simulink model "simLink_line"  (R2022b)
settings: Solver=FixedStepAuto  StartTime=0.0  StopTime=30  FixedStep=0.1  RelTol=1e-3
values from neighbouring files (symbols this model uses):
  length_body = pixel_body/pixel_conversion    (= 80)    [startSim.m]
  spacing = 2/pixel_conversion    (= 20)    [startSim.m]
undefined symbols (not defined in the file or in its folder): img, offset_x, offset_y, pixel, v1, v2
libraries: slpidlib x1, robotmobilelib x1
settings Model: Creator=andre  LastModifiedBy=andre

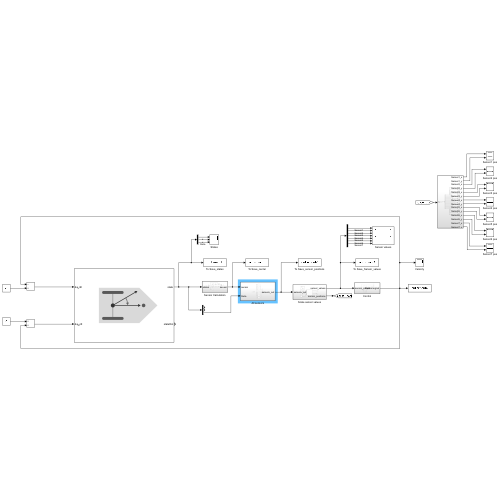
[thumbnail: Simulink's stored preview of the top-level diagram]
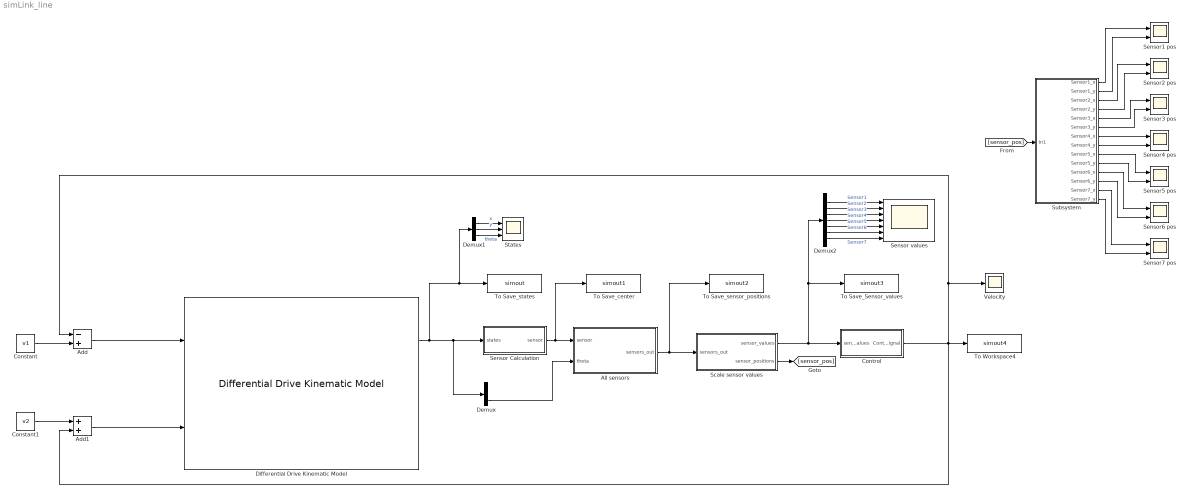
== system simLink_line ==
  Add : Sum  Inputs=-+
  Add1 : Sum
  All sensors : Subsystem
  Constant : Constant  Value=v1
  Constant1 : Constant  Value=v2
  Control : Subsystem
  Demux : Demux  Outputs=3
  Demux1 : Demux  Outputs=3
  Demux2 : Demux  Outputs=7
  Differential Drive Kinematic Model : robotmobilelib/Differential Drive Kinematic Model  VehicleInputs=Wheel Speeds  WheelRadius=0.5  WheelSpeedRange=[-inf inf]  TrackWidth=1  InitialState=initialState  SimulateUsing=Interpreted execution
  Scale sensor values : Subsystem
  Sensor Calculation : Subsystem
  Sensor values : Scope  NumInputPorts=7
  Sensor1 pos : Scope  NumInputPorts=2
  Sensor2 pos : Scope  NumInputPorts=2
  Sensor3 pos : Scope  NumInputPorts=2
  Sensor4 pos : Scope  NumInputPorts=2
  Sensor5 pos : Scope  NumInputPorts=2
  Sensor6 pos : Scope  NumInputPorts=2
  Sensor7 pos : Scope  NumInputPorts=2
  States : Scope  NumInputPorts=3
  Subsystem : Subsystem
  To Save_Sensor_values : ToWorkspace  VariableName=simout3  SaveFormat=Structure With Time  SampleTime=-1
  To Save_center : ToWorkspace  VariableName=simout1  SaveFormat=Structure With Time  SampleTime=-1
  To Save_sensor_positions : ToWorkspace  VariableName=simout2  SaveFormat=Structure With Time  SampleTime=-1
  To Save_states : ToWorkspace  VariableName=simout  SaveFormat=Structure With Time  SampleTime=-1
  To Workspace4 : ToWorkspace  VariableName=simout4  SaveFormat=Structure With Time  SampleTime=-1
  Velocity : Scope
  wires:
  Sensor Calculation/1(sensor) -> To Save_center/1, All sensors/1(sensor)
  Differential Drive Kinematic Model/1 -> Demux1/1, To Save_states/1, Demux/1, Sensor Calculation/1(states)
  All sensors/1(sensors_out) -> To Save_sensor_positions/1, Scale sensor values/1(sensors_out)
  Demux/3 -> All sensors/2(theta)
  Control/1(Control signal) -> Add1/2, To Workspace4/1, Add/1, Velocity/1
  Constant/1 -> Add/2
  Constant1/1 -> Add1/1
  Add1/1 -> Differential Drive Kinematic Model/2
  Add/1 -> Differential Drive Kinematic Model/1
  Demux1/1 -> States/1  "x"
  Demux1/2 -> States/2  "y"
  Demux1/3 -> States/3  "theta"
  Scale sensor values/1(sensor_values) -> Demux2/1, To Save_Sensor_values/1, Control/1(sensor_values)
  Demux2/1 -> Sensor values/1  "Sensor1"
  Demux2/2 -> Sensor values/2  "Sensor2"
  Demux2/3 -> Sensor values/3  "Sensor3"
  Demux2/4 -> Sensor values/4  "Sensor4"
  Demux2/5 -> Sensor values/5  "Sensor5"
  Demux2/6 -> Sensor values/6  "Sensor6"
  Demux2/7 -> Sensor values/7  "Sensor7"
  [sensor_pos] -> Subsystem/1(In1)
  Subsystem/1(Sensor1_x) -> Sensor1 pos/1
  Subsystem/2(Sensor1_y) -> Sensor1 pos/2
  Subsystem/3(Sensor2_x) -> Sensor2 pos/1
  Subsystem/4(Sensor2_y) -> Sensor2 pos/2
  Subsystem/5(Sensor3_x) -> Sensor3 pos/1
  Subsystem/6(Sensor3_y) -> Sensor3 pos/2
  Subsystem/7(Sensor4_x) -> Sensor4 pos/1
  Subsystem/8(Sensor4_y) -> Sensor4 pos/2
  Subsystem/9(Sensor5_x) -> Sensor5 pos/1
  Subsystem/10(Sensor5_y) -> Sensor5 pos/2
  Subsystem/11(Sensor6_x) -> Sensor6 pos/1
  Subsystem/12(Sensor6_y) -> Sensor6 pos/2
  Subsystem/13(Sensor7_x) -> Sensor7 pos/1
  Subsystem/14(Sensor7_y) -> Sensor7 pos/2
  Scale sensor values/2(sensor_positions) -> [sensor_pos]

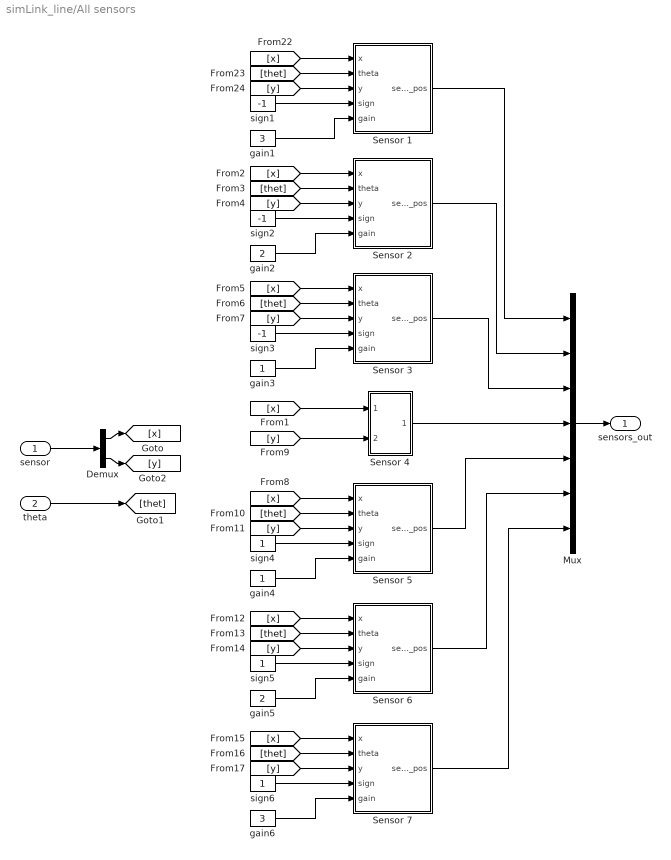
== system simLink_line/All sensors ==
  sensor : Inport
  theta : Inport  Port=2
  Demux : Demux  Outputs=2
  Mux : Mux  Inputs=7
  Sensor 1 : Subsystem
  Sensor 2 : Subsystem
  Sensor 3 : Subsystem
  Sensor 4 : Subsystem
  Sensor 5 : Subsystem
  Sensor 6 : Subsystem
  Sensor 7 : Subsystem
  gain1 : Constant  Value=3
  gain2 : Constant  Value=2
  gain3 : Constant
  gain4 : Constant
  gain5 : Constant  Value=2
  gain6 : Constant  Value=3
  sign1 : Constant  Value=-1
  sign2 : Constant  Value=-1
  sign3 : Constant  Value=-1
  sign4 : Constant
  sign5 : Constant
  sign6 : Constant
  sensors_out : Outport
  wires:
  sensor/1 -> Demux/1
  Demux/1 -> [x]
  theta/1 -> [thet]
  Demux/2 -> [y]
  Mux/1 -> sensors_out/1
  [x] -> Sensor 1/1(x)
  [thet] -> Sensor 1/2(theta)
  [y] -> Sensor 1/3(y)
  Sensor 1/1(sensor_pos) -> Mux/1
  [x] -> Sensor 4/1(In1)
  [y] -> Sensor 4/2(In2)
  Sensor 4/1(Out1) -> Mux/4
  sign1/1 -> Sensor 1/4(sign)
  gain1/1 -> Sensor 1/5(gain)
  [x] -> Sensor 2/1(x)
  [x] -> Sensor 3/1(x)
  [x] -> Sensor 5/1(x)
  [thet] -> Sensor 5/2(theta)
  [x] -> Sensor 6/1(x)
  [x] -> Sensor 7/1(x)
  Sensor 2/1(sensor_pos) -> Mux/2
  Sensor 3/1(sensor_pos) -> Mux/3
  Sensor 5/1(sensor_pos) -> Mux/5
  Sensor 6/1(sensor_pos) -> Mux/6
  Sensor 7/1(sensor_pos) -> Mux/7
  [thet] -> Sensor 2/2(theta)
  [y] -> Sensor 2/3(y)
  sign2/1 -> Sensor 2/4(sign)
  gain2/1 -> Sensor 2/5(gain)
  [thet] -> Sensor 3/2(theta)
  [y] -> Sensor 3/3(y)
  gain3/1 -> Sensor 3/5(gain)
  sign3/1 -> Sensor 3/4(sign)
  [y] -> Sensor 5/3(y)
  sign4/1 -> Sensor 5/4(sign)
  gain4/1 -> Sensor 5/5(gain)
  [thet] -> Sensor 6/2(theta)
  [y] -> Sensor 6/3(y)
  sign5/1 -> Sensor 6/4(sign)
  gain5/1 -> Sensor 6/5(gain)
  [thet] -> Sensor 7/2(theta)
  [y] -> Sensor 7/3(y)
  sign6/1 -> Sensor 7/4(sign)
  gain6/1 -> Sensor 7/5(gain)

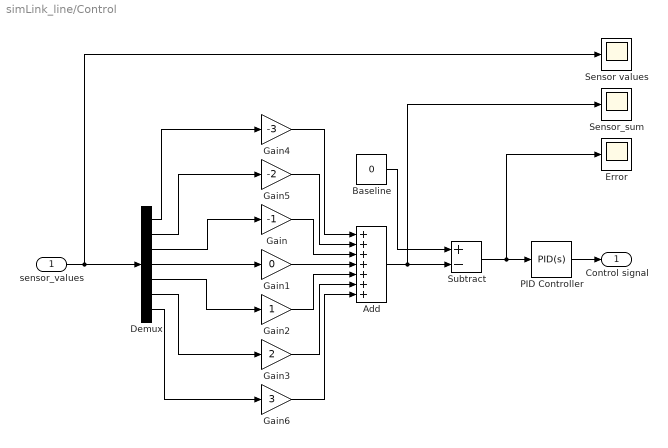
== system simLink_line/Control ==
  sensor_values : Inport
  Add : Sum  Inputs=+++++++
  Baseline : Constant  Value=0
  Demux : Demux  Outputs=7
  Error : Scope
  Gain : Gain  Gain=-1
  Gain1 : Gain  Gain=0
  Gain2 : Gain
  Gain3 : Gain  Gain=2
  Gain4 : Gain  Gain=-3
  Gain5 : Gain  Gain=-2
  Gain6 : Gain  Gain=3
  PID Controller : slpidlib/PID Controller  Controller=PID  Form=Parallel  TimeDomain=Continuous-time  UseExternalTs=off  SampleTime=-1  IntegratorMethod=Forward Euler  FilterMethod=Forward Euler  ControllerParametersSource=internal  P=0.01  I=1  UseKiTs=off  D=0  N=100  UseFilter=on  TunerSelectOption=Transfer Function Based (PID Tuner App)  InitialConditionSource=internal  InitialConditionForIntegrator=0  InitialConditionForFilter=0  DifferentiatorICPrevScaledInput=0  ExternalReset=none  TrackingMode=off  Kt=1  LimitOutput=off  SatLimitsSource=internal  UpperSaturationLimit=inf  LowerSaturationLimit=-inf  LinearizeAsGain=on  AntiWindupMode=none  Kb=1  LimitIntegrator=off  UpperIntegratorSaturationLimit=inf  LowerIntegratorSaturationLimit=-inf  POutMin=[]  POutMax=[]  IOutMin=[]  IOutMax=[]  DOutMin=[]  DOutMax=[]  NOutMin=[]  NOutMax=[]  SumOutMin=[]  SumOutMax=[]  SaturationOutMin=[]  SaturationOutMax=[]  PParamMin=[]  PParamMax=[]  IParamMin=[]  IParamMax=[]  DParamMin=[]  DParamMax=[]  NParamMin=[]  NParamMax=[]  KbParamMin=[]  KbParamMax=[]  KtParamMin=[]  KtParamMax=[]  KbOutMin=[]  KbOutMax=[]  KtOutMin=[]  KtOutMax=[]  IntegratorOutMin=[]  IntegratorOutMax=[]  FilterOutMin=[]  FilterOutMax=[]  SumI1OutMin=[]  SumI1OutMax=[]  SumI2OutMin=[]  SumI2OutMax=[]  SumI3OutMin=[]  SumI3OutMax=[]  SumI4OutMin=[]  SumI4OutMax=[]  SumDOutMin=[]  SumDOutMax=[]  DifferentiatorOutMin=[]  DifferentiatorOutMax=[]  FilterDiffOutCoefMin=[]  FilterDiffOutCoefMax=[]  ReciprocalOutMin=[]  ReciprocalOutMax=[]  SumDenOutMin=[]  SumDenOutMax=[]  SumNumOutMin=[]  SumNumOutMax=[]  DivideOutMin=[]  DivideOutMax=[]  UdiffTsProdOutMin=[]  UdiffTsProdOutMax=[]  NTsProdOutMin=[]  NTsProdOutMax=[]  UintegralTsProdOutMin=[]  UintegralTsProdOutMax=[]  UngainTsProdOutMin=[]  UngainTsProdOutMax=[]  ClampingZeroOutDataTypeStr=Inherit: Inherit via back propagation  ClampingZeroOutMin=[]  ClampingZeroOutMax=[]  FilterDenConstantOutDataTypeStr=Inherit: Inherit via back propagation  FilterDenConstantOutMin=[]  FilterDenConstantOutMax=[]  PCopyOutDataTypeStr=Inherit: Inherit via back propagation  PCopyOutMin=[]  PCopyOutMax=[]  NCopyOutDataTypeStr=Inherit: Inherit via back propagation  NCopyOutMin=[]  NCopyOutMax=[]  IntegratorContinuousStateAttributes=''  IntegratorStateMustResolveToSignalObject=off  IntegratorRTWStateStorageClass=Auto  FilterContinuousStateAttributes=''  FilterStateMustResolveToSignalObject=off  FilterRTWStateStorageClass=Auto  ParallelPVariant=InternalParameters  IdealPVariant=Disabled  IVariant=InternalParameters  DVariant=InternalParameters  IntegratorVariant=Continuous  SatVariant=Disabled  AWVariant=Passthrough  PCopyVariant=Disabled  TRVariant=Disabled  FdbkBlocksVariant=Forward  IdealPFdbkVariant=Disabled  SatFdbkVariant=Disabled  DerivativeFilterVariant=ContFilter  NVariant=InternalParameters  NCopyVariant=Disabled  FilterICVariant=InternalICsFilter  IntegratorICVariant=InternalICs  ExternalResetVariant=Disabled  TRSumVariant=Passthrough  SumFdbkVariant=Disabled  SumVariant=Sum_PID  TsampFilterVariant=InternalTs  TsampNgainVariant=Passthrough  TsampIntegralVariant=Passthrough  ExternalSaturationOutDataTypeStr=Inherit: Same as second input
  Sensor values : Scope
  Sensor_sum : Scope
  Subtract : Sum  Inputs=+-
  Control signal : Outport
  wires:
  sensor_values/1 -> Sensor values/1, Demux/1
  Baseline/1 -> Subtract/1
  Subtract/1 -> Error/1, PID Controller/1
  PID Controller/1 -> Control signal/1
  Gain4/1 -> Add/1
  Gain5/1 -> Add/2
  Gain/1 -> Add/3
  Gain1/1 -> Add/4
  Gain2/1 -> Add/5
  Gain3/1 -> Add/6
  Gain6/1 -> Add/7
  Demux/1 -> Gain4/1
  Demux/2 -> Gain5/1
  Demux/3 -> Gain/1
  Demux/4 -> Gain1/1
  Demux/5 -> Gain2/1
  Demux/6 -> Gain3/1
  Demux/7 -> Gain6/1
  Add/1 -> Sensor_sum/1, Subtract/2

== system simLink_line/Scale sensor values ==
  sensors_out : Inport
  Image : Constant  Value=img
  MATLAB Function : MATLAB Function  TreatAsAtomicUnit=on
  Offset for x : Constant  Value=offset_x
  Offset for y : Constant  Value=offset_y
  Pixel Size : Constant  Value=pixel
  sensor_values : Outport
  sensor_positions : Outport  Port=2
  wires:
  sensors_out/1 -> MATLAB Function/1(coord)
  MATLAB Function/1(sensor_values) -> sensor_values/1
  Image/1 -> MATLAB Function/2(img)
  Offset for x/1 -> MATLAB Function/3(offset_x)
  Offset for y/1 -> MATLAB Function/4(offset_y)
  Pixel Size/1 -> MATLAB Function/5(pixel)
  MATLAB Function/2(pos) -> sensor_positions/1

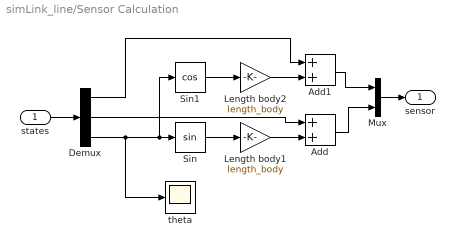
== system simLink_line/Sensor Calculation ==
  states : Inport
  Add : Sum
  Add1 : Sum
  Demux : Demux  Outputs=3
  Length body1 : Gain  Gain=length_body
  Length body2 : Gain  Gain=length_body
  Mux : Mux  Inputs=2
  Sin : Trigonometry
  Sin1 : Trigonometry  Operator=cos
  theta : Scope
  sensor : Outport
  wires:
  Mux/1 -> sensor/1
  Length body1/1 -> Add/2
  Demux/1 -> Add1/1
  Sin/1 -> Length body1/1
  Demux/3 -> theta/1, Sin1/1, Sin/1
  Length body2/1 -> Add1/2
  Sin1/1 -> Length body2/1
  Demux/2 -> Add/1
  states/1 -> Demux/1
  Add1/1 -> Mux/1
  Add/1 -> Mux/2

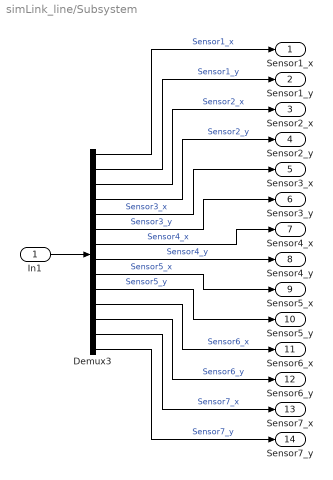
== system simLink_line/Subsystem ==
  In1 : Inport
  Demux3 : Demux  Outputs=14
  Sensor1_x : Outport
  Sensor1_y : Outport  Port=2
  Sensor2_x : Outport  Port=3
  Sensor2_y : Outport  Port=4
  Sensor3_x : Outport  Port=5
  Sensor3_y : Outport  Port=6
  Sensor4_x : Outport  Port=7
  Sensor4_y : Outport  Port=8
  Sensor5_x : Outport  Port=9
  Sensor5_y : Outport  Port=10
  Sensor6_x : Outport  Port=11
  Sensor6_y : Outport  Port=12
  Sensor7_x : Outport  Port=13
  Sensor7_y : Outport  Port=14
  wires:
  Demux3/5 -> Sensor3_x/1  "Sensor3_x"
  Demux3/3 -> Sensor2_x/1  "Sensor2_x"
  Demux3/7 -> Sensor4_x/1  "Sensor4_x"
  Demux3/8 -> Sensor4_y/1  "Sensor4_y"
  Demux3/12 -> Sensor6_y/1  "Sensor6_y"
  Demux3/4 -> Sensor2_y/1  "Sensor2_y"
  Demux3/1 -> Sensor1_x/1  "Sensor1_x"
  Demux3/13 -> Sensor7_x/1  "Sensor7_x"
  In1/1 -> Demux3/1
  Demux3/6 -> Sensor3_y/1  "Sensor3_y"
  Demux3/14 -> Sensor7_y/1  "Sensor7_y"
  Demux3/2 -> Sensor1_y/1  "Sensor1_y"
  Demux3/11 -> Sensor6_x/1  "Sensor6_x"
  Demux3/10 -> Sensor5_y/1  "Sensor5_y"
  Demux3/9 -> Sensor5_x/1  "Sensor5_x"

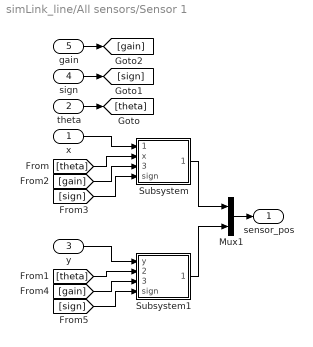
== system simLink_line/All sensors/Sensor 1 ==
  x : Inport
  theta : Inport  Port=2
  y : Inport  Port=3
  sign : Inport  Port=4
  gain : Inport  Port=5
  Mux1 : Mux  Inputs=2
  Subsystem : Subsystem
  Subsystem1 : Subsystem
  sensor_pos : Outport
  wires:
  x/1 -> Subsystem/1(theta)
  Mux1/1 -> sensor_pos/1
  Subsystem1/1(y_pos) -> Mux1/2
  Subsystem/1(x_pos) -> Mux1/1
  theta/1 -> [theta]
  y/1 -> Subsystem1/1(y)
  [theta] -> Subsystem/2(x)
  [theta] -> Subsystem1/2(theta)
  sign/1 -> [sign]
  gain/1 -> [gain]
  [gain] -> Subsystem/3(gain)
  [sign] -> Subsystem/4(sign)
  [gain] -> Subsystem1/3(gain)
  [sign] -> Subsystem1/4(sign)

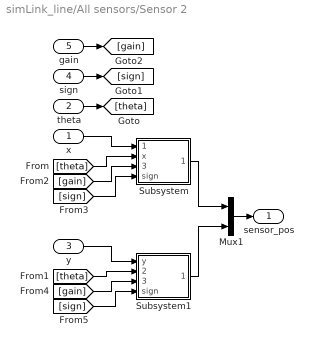
== system simLink_line/All sensors/Sensor 2 ==
  x : Inport
  theta : Inport  Port=2
  y : Inport  Port=3
  sign : Inport  Port=4
  gain : Inport  Port=5
  Mux1 : Mux  Inputs=2
  Subsystem : Subsystem
  Subsystem1 : Subsystem
  sensor_pos : Outport
  wires:
  x/1 -> Subsystem/1(theta)
  Mux1/1 -> sensor_pos/1
  Subsystem1/1(y_pos) -> Mux1/2
  Subsystem/1(x_pos) -> Mux1/1
  theta/1 -> [theta]
  y/1 -> Subsystem1/1(y)
  [theta] -> Subsystem/2(x)
  [theta] -> Subsystem1/2(theta)
  sign/1 -> [sign]
  gain/1 -> [gain]
  [gain] -> Subsystem/3(gain)
  [sign] -> Subsystem/4(sign)
  [gain] -> Subsystem1/3(gain)
  [sign] -> Subsystem1/4(sign)

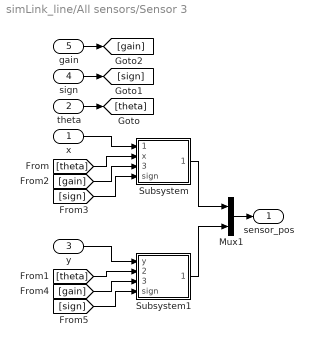
== system simLink_line/All sensors/Sensor 3 ==
  x : Inport
  theta : Inport  Port=2
  y : Inport  Port=3
  sign : Inport  Port=4
  gain : Inport  Port=5
  Mux1 : Mux  Inputs=2
  Subsystem : Subsystem
  Subsystem1 : Subsystem
  sensor_pos : Outport
  wires:
  x/1 -> Subsystem/1(theta)
  Mux1/1 -> sensor_pos/1
  Subsystem1/1(y_pos) -> Mux1/2
  Subsystem/1(x_pos) -> Mux1/1
  theta/1 -> [theta]
  y/1 -> Subsystem1/1(y)
  [theta] -> Subsystem/2(x)
  [theta] -> Subsystem1/2(theta)
  sign/1 -> [sign]
  gain/1 -> [gain]
  [gain] -> Subsystem/3(gain)
  [sign] -> Subsystem/4(sign)
  [gain] -> Subsystem1/3(gain)
  [sign] -> Subsystem1/4(sign)

== system simLink_line/All sensors/Sensor 4 ==
  In1 : Inport
  In2 : Inport  Port=2
  Mux4 : Mux  Inputs=2
  Out1 : Outport
  wires:
  In2/1 -> Mux4/2
  In1/1 -> Mux4/1
  Mux4/1 -> Out1/1

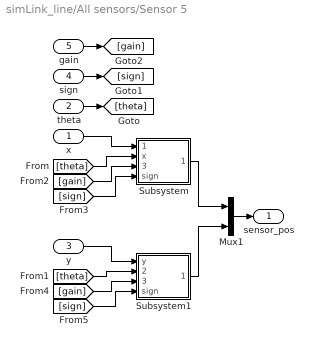
== system simLink_line/All sensors/Sensor 5 ==
  x : Inport
  theta : Inport  Port=2
  y : Inport  Port=3
  sign : Inport  Port=4
  gain : Inport  Port=5
  Mux1 : Mux  Inputs=2
  Subsystem : Subsystem
  Subsystem1 : Subsystem
  sensor_pos : Outport
  wires:
  x/1 -> Subsystem/1(theta)
  Mux1/1 -> sensor_pos/1
  Subsystem1/1(y_pos) -> Mux1/2
  Subsystem/1(x_pos) -> Mux1/1
  theta/1 -> [theta]
  y/1 -> Subsystem1/1(y)
  [theta] -> Subsystem/2(x)
  [theta] -> Subsystem1/2(theta)
  sign/1 -> [sign]
  gain/1 -> [gain]
  [gain] -> Subsystem/3(gain)
  [sign] -> Subsystem/4(sign)
  [gain] -> Subsystem1/3(gain)
  [sign] -> Subsystem1/4(sign)

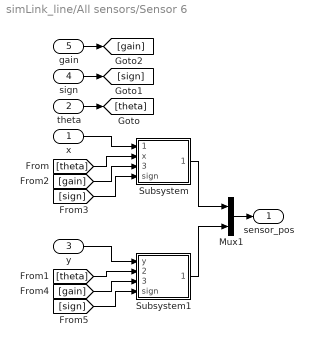
== system simLink_line/All sensors/Sensor 6 ==
  x : Inport
  theta : Inport  Port=2
  y : Inport  Port=3
  sign : Inport  Port=4
  gain : Inport  Port=5
  Mux1 : Mux  Inputs=2
  Subsystem : Subsystem
  Subsystem1 : Subsystem
  sensor_pos : Outport
  wires:
  x/1 -> Subsystem/1(theta)
  Mux1/1 -> sensor_pos/1
  Subsystem1/1(y_pos) -> Mux1/2
  Subsystem/1(x_pos) -> Mux1/1
  theta/1 -> [theta]
  y/1 -> Subsystem1/1(y)
  [theta] -> Subsystem/2(x)
  [theta] -> Subsystem1/2(theta)
  sign/1 -> [sign]
  gain/1 -> [gain]
  [gain] -> Subsystem/3(gain)
  [sign] -> Subsystem/4(sign)
  [gain] -> Subsystem1/3(gain)
  [sign] -> Subsystem1/4(sign)

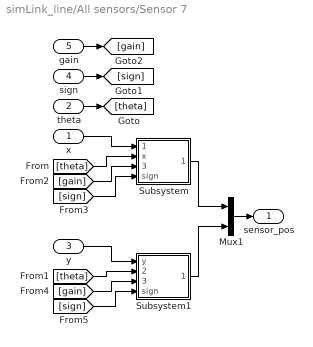
== system simLink_line/All sensors/Sensor 7 ==
  x : Inport
  theta : Inport  Port=2
  y : Inport  Port=3
  sign : Inport  Port=4
  gain : Inport  Port=5
  Mux1 : Mux  Inputs=2
  Subsystem : Subsystem
  Subsystem1 : Subsystem
  sensor_pos : Outport
  wires:
  x/1 -> Subsystem/1(theta)
  Mux1/1 -> sensor_pos/1
  Subsystem1/1(y_pos) -> Mux1/2
  Subsystem/1(x_pos) -> Mux1/1
  theta/1 -> [theta]
  y/1 -> Subsystem1/1(y)
  [theta] -> Subsystem/2(x)
  [theta] -> Subsystem1/2(theta)
  sign/1 -> [sign]
  gain/1 -> [gain]
  [gain] -> Subsystem/3(gain)
  [sign] -> Subsystem/4(sign)
  [gain] -> Subsystem1/3(gain)
  [sign] -> Subsystem1/4(sign)

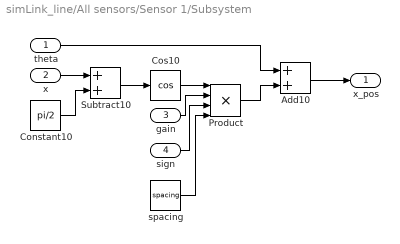
== system simLink_line/All sensors/Sensor 1/Subsystem ==
  theta : Inport
  x : Inport  Port=2
  gain : Inport  Port=3
  sign : Inport  Port=4
  Add10 : Sum
  Constant10 : Constant  Value=pi/2
  Cos10 : Trigonometry  Operator=cos
  Product : Product  Inputs=4
  Subtract10 : Sum
  spacing : Constant  Value=spacing
  x_pos : Outport
  wires:
  Subtract10/1 -> Cos10/1
  Add10/1 -> x_pos/1
  Constant10/1 -> Subtract10/2
  x/1 -> Subtract10/1
  theta/1 -> Add10/1
  Product/1 -> Add10/2
  Cos10/1 -> Product/1
  gain/1 -> Product/2
  sign/1 -> Product/3
  spacing/1 -> Product/4

== system simLink_line/All sensors/Sensor 1/Subsystem1 ==
  y : Inport
  theta : Inport  Port=2
  gain : Inport  Port=3
  sign : Inport  Port=4
  Add11 : Sum
  Constant11 : Constant  Value=pi/2
  Cos11 : Trigonometry
  Product : Product  Inputs=4
  Subtract11 : Sum
  spacing : Constant  Value=spacing
  y_pos : Outport
  wires:
  Subtract11/1 -> Cos11/1
  Constant11/1 -> Subtract11/2
  y/1 -> Add11/1
  Cos11/1 -> Product/1
  Add11/1 -> y_pos/1
  Product/1 -> Add11/2
  theta/1 -> Subtract11/1
  sign/1 -> Product/3
  gain/1 -> Product/2
  spacing/1 -> Product/4

== system simLink_line/All sensors/Sensor 2/Subsystem ==
  theta : Inport
  x : Inport  Port=2
  gain : Inport  Port=3
  sign : Inport  Port=4
  Add10 : Sum
  Constant10 : Constant  Value=pi/2
  Cos10 : Trigonometry  Operator=cos
  Product : Product  Inputs=4
  Subtract10 : Sum
  spacing : Constant  Value=spacing
  x_pos : Outport
  wires:
  Subtract10/1 -> Cos10/1
  Add10/1 -> x_pos/1
  Constant10/1 -> Subtract10/2
  x/1 -> Subtract10/1
  theta/1 -> Add10/1
  Product/1 -> Add10/2
  Cos10/1 -> Product/1
  gain/1 -> Product/2
  sign/1 -> Product/3
  spacing/1 -> Product/4

== system simLink_line/All sensors/Sensor 2/Subsystem1 ==
  y : Inport
  theta : Inport  Port=2
  gain : Inport  Port=3
  sign : Inport  Port=4
  Add11 : Sum
  Constant11 : Constant  Value=pi/2
  Cos11 : Trigonometry
  Product : Product  Inputs=4
  Subtract11 : Sum
  spacing : Constant  Value=spacing
  y_pos : Outport
  wires:
  Subtract11/1 -> Cos11/1
  Constant11/1 -> Subtract11/2
  y/1 -> Add11/1
  Cos11/1 -> Product/1
  Add11/1 -> y_pos/1
  Product/1 -> Add11/2
  theta/1 -> Subtract11/1
  sign/1 -> Product/3
  gain/1 -> Product/2
  spacing/1 -> Product/4

== system simLink_line/All sensors/Sensor 3/Subsystem ==
  theta : Inport
  x : Inport  Port=2
  gain : Inport  Port=3
  sign : Inport  Port=4
  Add10 : Sum
  Constant10 : Constant  Value=pi/2
  Cos10 : Trigonometry  Operator=cos
  Product : Product  Inputs=4
  Subtract10 : Sum
  spacing : Constant  Value=spacing
  x_pos : Outport
  wires:
  Subtract10/1 -> Cos10/1
  Add10/1 -> x_pos/1
  Constant10/1 -> Subtract10/2
  x/1 -> Subtract10/1
  theta/1 -> Add10/1
  Product/1 -> Add10/2
  Cos10/1 -> Product/1
  gain/1 -> Product/2
  sign/1 -> Product/3
  spacing/1 -> Product/4

== system simLink_line/All sensors/Sensor 3/Subsystem1 ==
  y : Inport
  theta : Inport  Port=2
  gain : Inport  Port=3
  sign : Inport  Port=4
  Add11 : Sum
  Constant11 : Constant  Value=pi/2
  Cos11 : Trigonometry
  Product : Product  Inputs=4
  Subtract11 : Sum
  spacing : Constant  Value=spacing
  y_pos : Outport
  wires:
  Subtract11/1 -> Cos11/1
  Constant11/1 -> Subtract11/2
  y/1 -> Add11/1
  Cos11/1 -> Product/1
  Add11/1 -> y_pos/1
  Product/1 -> Add11/2
  theta/1 -> Subtract11/1
  sign/1 -> Product/3
  gain/1 -> Product/2
  spacing/1 -> Product/4

== system simLink_line/All sensors/Sensor 5/Subsystem ==
  theta : Inport
  x : Inport  Port=2
  gain : Inport  Port=3
  sign : Inport  Port=4
  Add10 : Sum
  Constant10 : Constant  Value=pi/2
  Cos10 : Trigonometry  Operator=cos
  Product : Product  Inputs=4
  Subtract10 : Sum
  spacing : Constant  Value=spacing
  x_pos : Outport
  wires:
  Subtract10/1 -> Cos10/1
  Add10/1 -> x_pos/1
  Constant10/1 -> Subtract10/2
  x/1 -> Subtract10/1
  theta/1 -> Add10/1
  Product/1 -> Add10/2
  Cos10/1 -> Product/1
  gain/1 -> Product/2
  sign/1 -> Product/3
  spacing/1 -> Product/4

== system simLink_line/All sensors/Sensor 5/Subsystem1 ==
  y : Inport
  theta : Inport  Port=2
  gain : Inport  Port=3
  sign : Inport  Port=4
  Add11 : Sum
  Constant11 : Constant  Value=pi/2
  Cos11 : Trigonometry
  Product : Product  Inputs=4
  Subtract11 : Sum
  spacing : Constant  Value=spacing
  y_pos : Outport
  wires:
  Subtract11/1 -> Cos11/1
  Constant11/1 -> Subtract11/2
  y/1 -> Add11/1
  Cos11/1 -> Product/1
  Add11/1 -> y_pos/1
  Product/1 -> Add11/2
  theta/1 -> Subtract11/1
  sign/1 -> Product/3
  gain/1 -> Product/2
  spacing/1 -> Product/4

== system simLink_line/All sensors/Sensor 6/Subsystem ==
  theta : Inport
  x : Inport  Port=2
  gain : Inport  Port=3
  sign : Inport  Port=4
  Add10 : Sum
  Constant10 : Constant  Value=pi/2
  Cos10 : Trigonometry  Operator=cos
  Product : Product  Inputs=4
  Subtract10 : Sum
  spacing : Constant  Value=spacing
  x_pos : Outport
  wires:
  Subtract10/1 -> Cos10/1
  Add10/1 -> x_pos/1
  Constant10/1 -> Subtract10/2
  x/1 -> Subtract10/1
  theta/1 -> Add10/1
  Product/1 -> Add10/2
  Cos10/1 -> Product/1
  gain/1 -> Product/2
  sign/1 -> Product/3
  spacing/1 -> Product/4

== system simLink_line/All sensors/Sensor 6/Subsystem1 ==
  y : Inport
  theta : Inport  Port=2
  gain : Inport  Port=3
  sign : Inport  Port=4
  Add11 : Sum
  Constant11 : Constant  Value=pi/2
  Cos11 : Trigonometry
  Product : Product  Inputs=4
  Subtract11 : Sum
  spacing : Constant  Value=spacing
  y_pos : Outport
  wires:
  Subtract11/1 -> Cos11/1
  Constant11/1 -> Subtract11/2
  y/1 -> Add11/1
  Cos11/1 -> Product/1
  Add11/1 -> y_pos/1
  Product/1 -> Add11/2
  theta/1 -> Subtract11/1
  sign/1 -> Product/3
  gain/1 -> Product/2
  spacing/1 -> Product/4

== system simLink_line/All sensors/Sensor 7/Subsystem ==
  theta : Inport
  x : Inport  Port=2
  gain : Inport  Port=3
  sign : Inport  Port=4
  Add10 : Sum
  Constant10 : Constant  Value=pi/2
  Cos10 : Trigonometry  Operator=cos
  Product : Product  Inputs=4
  Subtract10 : Sum
  spacing : Constant  Value=spacing
  x_pos : Outport
  wires:
  Subtract10/1 -> Cos10/1
  Add10/1 -> x_pos/1
  Constant10/1 -> Subtract10/2
  x/1 -> Subtract10/1
  theta/1 -> Add10/1
  Product/1 -> Add10/2
  Cos10/1 -> Product/1
  gain/1 -> Product/2
  sign/1 -> Product/3
  spacing/1 -> Product/4

== system simLink_line/All sensors/Sensor 7/Subsystem1 ==
  y : Inport
  theta : Inport  Port=2
  gain : Inport  Port=3
  sign : Inport  Port=4
  Add11 : Sum
  Constant11 : Constant  Value=pi/2
  Cos11 : Trigonometry
  Product : Product  Inputs=4
  Subtract11 : Sum
  spacing : Constant  Value=spacing
  y_pos : Outport
  wires:
  Subtract11/1 -> Cos11/1
  Constant11/1 -> Subtract11/2
  y/1 -> Add11/1
  Cos11/1 -> Product/1
  Add11/1 -> y_pos/1
  Product/1 -> Add11/2
  theta/1 -> Subtract11/1
  sign/1 -> Product/3
  gain/1 -> Product/2
  spacing/1 -> Product/4

== matlab function simLink_line/Scale sensor values/MATLAB Function ==
  data: coord input; sensor_values output; img input; offset_x input; offset_y input; pixel input; pos output
function [sensor_values, pos] = fcn(coord, img, offset_x,offset_y, pixel)

sensor_values = zeros(7,1);
sensor_ones = ones(pixel*2+1,pixel*2+1);
pos = zeros(14,1);


x1 = round(coord(1) + offset_x);
y1 = round(coord(2) + offset_y);
x2 = round(coord(3) + offset_x);
y2 = round(coord(4) + offset_y);
x3 = round(coord(5) + offset_x);
y3 = round(coord(6) + offset_y);
x4 = round(coord(7) + offset_x);
y4 = round(coord(8) + offset_y);
x5 = round(coord(9) + offset_x);
y5 = round(coord(10) + offset_y);
x6 = round(coord(11) + offset_x);
y6 = round(coord(12) + offset_y);
x7 = round(coord(13) + offset_x);
y7 = round(coord(14) + offset_y);

sens1 = img(y1 - pixel:y1 + pixel, x1 - pixel:x1 + pixel);
sens2 = img(y2 - pixel:y2 + pixel, x2 - pixel:x2 + pixel);
sens3 = img(y3 - pixel:y3 + pixel, x3 - pixel:x3 + pixel);
sens4 = img(y4 - pixel:y4 + pixel, x4 - pixel:x4 + pixel);
sens5 = img(y5 - pixel:y5 + pixel, x5 - pixel:x5 + pixel);
sens6 = img(y6 - pixel:y6 + pixel, x6 - pixel:x6 + pixel);
sens7 = img(y7 - pixel:y7 + pixel, x7 - pixel:x7 + pixel);

sensor_values(1) = sum(dot(sens1, sensor_ones),2);
sensor_values(2) = sum(dot(sens2, sensor_ones),2);
sensor_values(3) = sum(dot(sens3, sensor_ones),2);
sensor_values(4) = sum(dot(sens4, sensor_ones),2);
sensor_values(5) = sum(dot(sens5, sensor_ones),2);
sensor_values(6) = sum(dot(sens6, sensor_ones),2);
sensor_values(7) = sum(dot(sens7, sensor_ones),2);

pos(1) = x1;
pos(2) = y1;
pos(3) = x2;
pos(4) = y2;
pos(5) = x3;
pos(6) = y3;
pos(7) = x4;
pos(8) = y4;
pos(9) = x5;
pos(10) = y5;
pos(11) = x6;
pos(12) = y6;
pos(13) = x7;
pos(14) = y7;
